simulink model "sampleModel2120_pp"  (R2021a)
settings: Solver=VariableStepAuto  StartTime=0.0  StopTime=10.0  RelTol=1e-3
undefined symbols (not defined in the file or in its folder): DiscIntNeverNeededParam, magnitude, Newton, Raphson
libraries: simulink x67, pid_lib x12
(part 3 of 3)

== system sampleModel2120_pp/cfblk57/cfblk12 ==
  cfblk1 : Inport
  cfblk8 : Inport  Port=2
  cfblk3 : simulink/Discrete/Tapped Delay  vinit=0.0  samptime=-1  NumDelays=1  DelayOrder=Oldest  includeCurrent=off
  cfblk4 : Delay  DelayLengthSource=Input port  SampleTime=1
      settings: InputPortMap=u0,p1
  cfblk5 : Rounding
  cfblk6 : Sin  TimeSource=Use external signal  SampleTime=0
  cfblk7 : Bias  Bias=[-951001195.400587]
  cyemi_{496..501} (6 alike) : DataTypeConversion  OutDataTypeStr=double
  cfblk2 : Outport
  cfblk9 : Outport  Port=2
  wires:
  cfblk7/1 -> cfblk2/1
  cfblk5/1 -> cyemi_496/1, cyemi_498/1
  cfblk4/1 -> cfblk9/1
  cyemi_496/1 -> cfblk3/1
  cyemi_497/1 -> cfblk4/1
  cfblk6/1 -> cyemi_497/1
  cyemi_498/1 -> cfblk4/2
  cyemi_499/1 -> cfblk5/1
  cfblk1/1 -> cyemi_499/1
  cyemi_500/1 -> cfblk6/1
  cfblk3/1 -> cyemi_500/1
  cyemi_501/1 -> cfblk7/1
  cfblk8/1 -> cyemi_501/1

== system sampleModel2120_pp/cfblk57/cfblk13 ==
  cfblk1 : Inport
  cfblk7 : Inport  Port=2
  cfblk3 : simulink/Discrete/Transfer Fcn Real Zero  ZeroZ=0.75  ICPrevInput=0.0  DoSatur=off
      settings: SourceProductBaseCode=SL
  cfblk4 : Sum  Inputs=+-  OutDataTypeStr=double
  cfblk5 : Signum
  cfblk6 : Squeeze
  cyemi_{504..507} (4 alike) : DataTypeConversion  OutDataTypeStr=double
  cfblk2 : Outport
  wires:
  cfblk3/1 -> cfblk6/1
  cfblk6/1 -> cfblk2/1, cyemi_507/1
  cyemi_504/1 -> cfblk3/1
  cfblk4/1 -> cyemi_504/1
  cyemi_505/1 -> cfblk4/1
  cfblk1/1 -> cyemi_505/1
  cyemi_506/1 -> cfblk4/2
  cfblk7/1 -> cyemi_506/1
  cyemi_507/1 -> cfblk5/1

== system sampleModel2120_pp/cfblk57/cfblk14 ==
  cfblk1 : Inport
  cfblk6 : Inport  Port=2
  cfblk3 : Gain  Gain=[374890354.692374]  OutDataTypeStr=double
  cfblk4 : Sqrt  Operator=rSqrt  OutDataTypeStr=double  AlgorithmType=Newton-Raphson  SaturateOnIntegerOverflow=on
  cfblk5 : Product  Inputs=*  OutDataTypeStr=double
  cyemi_510 : DataTypeConversion  OutDataTypeStr=double
  cyemi_511 : DataTypeConversion  OutDataTypeStr=double
  cyemi_512 : DataTypeConversion  OutDataTypeStr=double
  cfblk2 : Outport
  cfblk7 : Outport  Port=2
  cfblk8 : Outport  Port=3
  wires:
  cfblk3/1 -> cfblk7/1
  cfblk1/1 -> cfblk8/1, cyemi_512/1
  cfblk4/1 -> cfblk2/1
  cyemi_510/1 -> cfblk3/1
  cfblk6/1 -> cyemi_510/1
  cyemi_511/1 -> cfblk4/1
  cfblk5/1 -> cyemi_511/1
  cyemi_512/1 -> cfblk5/1

== system sampleModel2120_pp/cfblk57/cfblk15 ==
  cfblk1 : Inport
  cfblk13 : Inport  Port=2
  cfblk14 : Inport  Port=3
  cfblk15 : Inport  Port=4
  cfblk10 : Sin  TimeSource=Use external signal  SampleTime=0
  cfblk11 : UnaryMinus
  cfblk12 : Constant  Value=[495800150.814714]  OutDataTypeStr=double  SampleTime=1
  cfblk3 : simulink/Discrete/Transfer Fcn Real Zero  ZeroZ=0.75  ICPrevInput=0.0  DoSatur=off
      settings: SourceProductBaseCode=SL
  cfblk4 : DiscreteFilter  SampleTime=1
  cfblk5 : simulink/Discrete/Difference  ICPrevInput=0.0  OutMin=[]  OutMax=[]  OutDataTypeStr=double  OutputDataTypeScalingMode=double  OutDataType=fixdt(1, 16)  OutScaling=2^-10  DoSatur=off
  cfblk6 : simulink/Discrete/Transfer Fcn First Order  PoleZ=0.95  ICPrevOutput=0.0  DoSatur=off
  cfblk7 : UnaryMinus
  cfblk8 : MinMax  Inputs=3  OutDataTypeStr=double
  cfblk9 : DotProduct  OutDataTypeStr=double  InputSameDT=on
  cyemi_{517..528} (12 alike) : DataTypeConversion  OutDataTypeStr=double
  cfblk2 : Outport
  cfblk16 : Outport  Port=2
  cfblk17 : Outport  Port=3
  wires:
  cfblk8/1 -> cfblk16/1
  cfblk13/1 -> cfblk2/1
  cfblk10/1 -> cyemi_520/1, cyemi_521/1
  cfblk3/1 -> cfblk17/1
  cyemi_517/1 -> cfblk10/1
  cfblk1/1 -> cyemi_517/1
  cyemi_518/1 -> cfblk11/1
  cfblk15/1 -> cyemi_518/1
  cyemi_519/1 -> cfblk3/1
  cfblk5/1 -> cyemi_519/1
  cyemi_520/1 -> cfblk4/1
  cyemi_521/1 -> cfblk5/1
  cyemi_522/1 -> cfblk6/1
  cfblk9/1 -> cyemi_522/1
  cyemi_523/1 -> cfblk7/1
  cfblk4/1 -> cyemi_523/1
  cyemi_524/1 -> cfblk8/1
  cfblk14/1 -> cyemi_524/1
  cyemi_525/1 -> cfblk8/2
  cfblk6/1 -> cyemi_525/1
  cyemi_526/1 -> cfblk8/3
  cfblk12/1 -> cyemi_526/1
  cyemi_527/1 -> cfblk9/1
  cfblk11/1 -> cyemi_527/1
  cyemi_528/1 -> cfblk9/2
  cfblk7/1 -> cyemi_528/1

== system sampleModel2120_pp/cfblk57/cfblk16 ==
  cfblk1 : Inport
  cfblk13 : Inport  Port=2
  cfblk14 : Inport  Port=3
  cfblk15 : Inport  Port=4
  cfblk16 : Inport  Port=5
  cfblk10 : Abs  OutDataTypeStr=double
  cfblk11 : Sin  TimeSource=Use external signal  SampleTime=0
  cfblk12 : Constant  Value=[868731902.486093]  OutDataTypeStr=double  SampleTime=1
  cfblk3 : simulink/Discrete/Transfer Fcn Real Zero  ZeroZ=0.75  ICPrevInput=0.0  DoSatur=off
      settings: SourceProductBaseCode=SL
  cfblk4 : UnitDelay  HasFrameUpgradeWarning=on
  cfblk5 : Delay  SampleTime=1
  cfblk6 : Trigonometry
  cfblk7 : Sum  Inputs=+-  OutDataTypeStr=double
  cfblk8 : DotProduct  OutDataTypeStr=double  InputSameDT=on
  cfblk9 : Polyval  Coefs=[ +2.081618890e-019, -1.441693666e-014, +4.719686976e-010, -8.536869453e-006, +1.621573104e-001, -8.087801117e+001 ]
  cyemi_{534..544} (11 alike) : DataTypeConversion  OutDataTypeStr=double
  cfblk2 : Outport
  wires:
  cfblk8/1 -> cfblk2/1
  cyemi_534/1 -> cfblk10/1
  cfblk5/1 -> cyemi_534/1
  cyemi_535/1 -> cfblk11/1
  cfblk1/1 -> cyemi_535/1
  cyemi_536/1 -> cfblk3/1
  cfblk4/1 -> cyemi_536/1
  cyemi_537/1 -> cfblk4/1
  cfblk9/1 -> cyemi_537/1
  cyemi_538/1 -> cfblk5/1
  cfblk14/1 -> cyemi_538/1
  cyemi_539/1 -> cfblk6/1
  cfblk11/1 -> cyemi_539/1
  cyemi_540/1 -> cfblk7/1
  cfblk16/1 -> cyemi_540/1
  cyemi_541/1 -> cfblk7/2
  cfblk12/1 -> cyemi_541/1
  cyemi_542/1 -> cfblk8/1
  cfblk7/1 -> cyemi_542/1
  cyemi_543/1 -> cfblk8/2
  cfblk10/1 -> cyemi_543/1
  cyemi_544/1 -> cfblk9/1
  cfblk15/1 -> cyemi_544/1

== system sampleModel2120_pp/cfblk57/cfblk8 ==
  cfblk1 : Inport
  cfblk12 : Inport  Port=2
  cfblk13 : Inport  Port=3
  cfblk10 : Constant  Value=[-135185284.316877]  OutDataTypeStr=double  SampleTime=1
  cfblk11 : Constant  Value=[742840417.275004]  OutDataTypeStr=double  SampleTime=1
  cfblk14 : Delay  SampleTime=1
  cfblk3 : simulink/Discrete/Transfer Fcn Real Zero  ZeroZ=0.75  ICPrevInput=0.0  DoSatur=off
      settings: SourceProductBaseCode=SL
  cfblk4 : simulink/Discrete/Transfer Fcn Real Zero  ZeroZ=0.75  ICPrevInput=0.0  DoSatur=off
      settings: SourceProductBaseCode=SL
  cfblk5 : Delay  ShowEnablePort=on  SampleTime=1
      settings: InputPortMap=u0,e6
  cfblk6 : UnitDelay  HasFrameUpgradeWarning=on
  cfblk7 : Signum
  cfblk8 : DotProduct  OutDataTypeStr=double  InputSameDT=on
  cfblk9 : DotProduct  OutDataTypeStr=double  InputSameDT=on
  cyemi_{558..568} (11 alike) : DataTypeConversion  OutDataTypeStr=double
  cfblk2 : Outport
  wires:
  cfblk12/1 -> cfblk2/1
  cyemi_558/1 -> cfblk14/1
  cfblk8/1 -> cyemi_558/1
  cyemi_559/1 -> cfblk3/1
  cfblk14/1 -> cyemi_559/1
  cyemi_560/1 -> cfblk4/1
  cfblk6/1 -> cyemi_560/1
  cyemi_561/1 -> cfblk5/1
  cfblk1/1 -> cyemi_561/1
  cyemi_562/1 -> cfblk5/2
  cfblk7/1 -> cyemi_562/1
  cyemi_563/1 -> cfblk6/1
  cfblk11/1 -> cyemi_563/1
  cyemi_564/1 -> cfblk7/1
  cfblk13/1 -> cyemi_564/1
  cyemi_565/1 -> cfblk8/1
  cfblk3/1 -> cyemi_565/1
  cyemi_566/1 -> cfblk8/2
  cfblk9/1 -> cyemi_566/1
  cyemi_567/1 -> cfblk9/1
  cfblk4/1 -> cyemi_567/1
  cyemi_568/1 -> cfblk9/2
  cfblk10/1 -> cyemi_568/1

== system sampleModel2120_pp/cfblk57/cfblk9 ==
  cfblk1 : Inport
  cfblk6 : Inport  Port=2
  cfblk3 : DiscreteFilter  SampleTime=1
  cfblk4 : Sqrt  OutDataTypeStr=double  SaturateOnIntegerOverflow=on
  cfblk5 : Constant  Value=[-633278511.677385]  OutDataTypeStr=double  SampleTime=1
  cyemi_571 : DataTypeConversion  OutDataTypeStr=double
  cyemi_572 : DataTypeConversion  OutDataTypeStr=double
  cfblk2 : Outport
  cfblk7 : Outport  Port=2
  wires:
  cfblk4/1 -> cfblk7/1
  cfblk3/1 -> cfblk2/1
  cyemi_571/1 -> cfblk3/1
  cfblk6/1 -> cyemi_571/1
  cyemi_572/1 -> cfblk4/1
  cfblk5/1 -> cyemi_572/1

== system sampleModel2120_pp/cfblk60/cfblk13 ==
  cfblk1 : Inport
  cfblk7 : Inport  Port=2
  cfblk8 : Inport  Port=3
  cfblk9 : Inport  Port=4
  cfblk10 : Delay
  cfblk3 : DotProduct  OutDataTypeStr=double  InputSameDT=on
  cfblk4 : PermuteDimensions
  cfblk5 : DotProduct  OutDataTypeStr=double  InputSameDT=on
  cfblk6 : Signum
  cyemi_{584..590} (7 alike) : DataTypeConversion  OutDataTypeStr=double
  cfblk2 : Outport
  wires:
  cfblk7/1 -> cfblk2/1
  cyemi_584/1 -> cfblk10/1
  cfblk3/1 -> cyemi_584/1
  cyemi_585/1 -> cfblk3/1
  cfblk9/1 -> cyemi_585/1
  cyemi_586/1 -> cfblk3/2
  cfblk4/1 -> cyemi_586/1
  cyemi_587/1 -> cfblk4/1
  cfblk5/1 -> cyemi_587/1
  cyemi_588/1 -> cfblk5/1
  cfblk10/1 -> cyemi_588/1
  cyemi_589/1 -> cfblk5/2
  cfblk1/1 -> cyemi_589/1
  cyemi_590/1 -> cfblk6/1
  cfblk8/1 -> cyemi_590/1

== system sampleModel2120_pp/cfblk61/cfblk10 ==
  cfblk1 : Inport
  cfblk8 : Inport  Port=2
  cfblk9 : Inport  Port=3
  cfblk10 : Inport  Port=4
  cfblk3 : simulink/Discrete/Difference  ICPrevInput=0.0  OutMin=[]  OutMax=[]  OutDataTypeStr=double  OutputDataTypeScalingMode=double  OutDataType=fixdt(1, 16)  OutScaling=2^-10  DoSatur=off
  cfblk4 : pid_lib/PID Controller (2DOF)  Controller=PID  Form=Parallel  TimeDomain=Discrete-time  UseExternalTs=off  SampleTime=-1  IntegratorMethod=Forward Euler  FilterMethod=Forward Euler  ControllerParametersSource=internal  P=1  I=1  D=0  UseFilter=on  N=100  b=1  c=1  TunerSelectOption=Transfer Function Based (PID Tuner App)  InitialConditionSource=internal  InitialConditionForIntegrator=0  InitialConditionForFilter=0  DifferentiatorICPrevScaledInput=0  ExternalReset=none  TrackingMode=off  Kt=1  LimitOutput=off  SatLimitsSource=internal  UpperSaturationLimit=inf  LowerSaturationLimit=-inf  LinearizeAsGain=off  AntiWindupMode=none  Kb=1  POutMin=[]  POutMax=[]  IOutMin=[]  IOutMax=[]  DOutMin=[]  DOutMax=[]  NOutMin=[]  NOutMax=[]  bOutMin=[]  bOutMax=[]  cOutMin=[]  cOutMax=[]  SumOutMin=[]  SumOutMax=[]  SaturationOutMin=[]  SaturationOutMax=[]  PParamMin=[]  PParamMax=[]  IParamMin=[]  IParamMax=[]  DParamMin=[]  DParamMax=[]  NParamMin=[]  NParamMax=[]  bParamMin=[]  bParamMax=[]  cParamMin=[]  cParamMax=[]  KbParamMin=[]  KbParamMax=[]  KtParamMin=[]  KtParamMax=[]  KbOutMin=[]  KbOutMax=[]  KtOutMin=[]  KtOutMax=[]  IntegratorOutMin=[]  IntegratorOutMax=[]  FilterOutMin=[]  FilterOutMax=[]  SumI1OutMin=[]  SumI1OutMax=[]  SumI2OutMin=[]  SumI2OutMax=[]  SumI3OutMin=[]  SumI3OutMax=[]  SumI4OutMin=[]  SumI4OutMax=[]  SumDOutMin=[]  SumDOutMax=[]  Sum1OutMin=[]  Sum1OutMax=[]  Sum2OutMin=[]  Sum2OutMax=[]  Sum3OutMin=[]  Sum3OutMax=[]  DifferentiatorOutMin=[]  DifferentiatorOutMax=[]  FilterDiffOutCoefMin=[]  FilterDiffOutCoefMax=[]  ReciprocalOutMin=[]  ReciprocalOutMax=[]  SumDenOutMin=[]  SumDenOutMax=[]  SumNumOutMin=[]  SumNumOutMax=[]  DivideOutMin=[]  DivideOutMax=[]  UdiffTsProdOutMin=[]  UdiffTsProdOutMax=[]  NTsProdOutMin=[]  NTsProdOutMax=[]  UintegralTsProdOutMin=[]  UintegralTsProdOutMax=[]  UngainTsProdOutMin=[]  UngainTsProdOutMax=[]  IntegratorContinuousStateAttributes=''  IntegratorStateMustResolveToSignalObject=off  IntegratorRTWStateStorageClass=Auto  FilterContinuousStateAttributes=''  FilterStateMustResolveToSignalObject=off  FilterRTWStateStorageClass=Auto  ParallelPVariant=InternalParameters  IdealPVariant=Disabled  IVariant=InternalParameters  DVariant=InternalParameters  bVariant=InternalParameters  cVariant=InternalParameters  IntegratorVariant=Discrete  SatVariant=Disabled  AWVariant=Passthrough  PCopyVariant=Disabled  TRVariant=Disabled  FdbkBlocksVariant=Forward  IdealPFdbkVariant=Disabled  SatFdbkVariant=Disabled  DerivativeFilterVariant=ForwardEulerFilter  NVariant=InternalParameters  NCopyVariant=Disabled  FilterICVariant=InternalICsFilter  IntegratorICVariant=InternalICs  ExternalResetVariant=Disabled  TRSumVariant=Passthrough  SumFdbkVariant=Disabled  SumVariant=Sum_PID  TsampFilterVariant=InternalTs  TsampNgainVariant=Passthrough  TsampIntegralVariant=Passthrough  ExternalSaturationOutDataTypeStr=Inherit: Same as second input
      settings: SourceProductBaseCode=SL
  cfblk5 : Math  Operator=rem  OutDataTypeStr=double  SaturateOnIntegerOverflow=on
  cfblk6 : Constant  Value=[-573577766.807925]  OutDataTypeStr=double  SampleTime=1
  cfblk7 : Constant  Value=[290213308.563316]  OutDataTypeStr=double  SampleTime=1
  cyemi_{612..616} (5 alike) : DataTypeConversion  OutDataTypeStr=double
  cfblk2 : Outport
  wires:
  cfblk3/1 -> cfblk2/1
  cyemi_612/1 -> cfblk3/1
  cfblk8/1 -> cyemi_612/1
  cyemi_613/1 -> cfblk4/1
  cfblk1/1 -> cyemi_613/1
  cyemi_614/1 -> cfblk4/2
  cfblk10/1 -> cyemi_614/1
  cyemi_615/1 -> cfblk5/1
  cfblk9/1 -> cyemi_615/1
  cyemi_616/1 -> cfblk5/2
  cfblk7/1 -> cyemi_616/1

== system sampleModel2120_pp/cfblk61/cfblk11 ==
  cfblk1 : Inport
  cfblk3 : DiscreteTransferFcn
  cfblk4 : DiscreteFir
  cfblk5 : simulink/Discrete/Transfer Fcn Lead or Lag  PoleZ=0.95  ZeroZ=0.75  ICPrevOutput=0.0  ICPrevInput=0.0  DoSatur=off
      settings: SourceProductBaseCode=SL
  cfblk6 : MinMax  Inputs=3  OutDataTypeStr=double
  cfblk8 : Delay
  cyemi_{618..624} (7 alike) : DataTypeConversion  OutDataTypeStr=double
  cfblk2 : Outport
  cfblk7 : Outport  Port=2
  wires:
  cfblk6/1 -> cfblk2/1
  cfblk3/1 -> cfblk7/1, cyemi_622/1
  cfblk4/1 -> cyemi_620/1, cyemi_623/1
  cfblk1/1 -> cyemi_618/1, cyemi_621/1
  cyemi_618/1 -> cfblk3/1
  cyemi_619/1 -> cfblk4/1
  cfblk8/1 -> cyemi_619/1
  cyemi_620/1 -> cfblk5/1
  cyemi_621/1 -> cfblk6/1
  cyemi_622/1 -> cfblk6/2
  cyemi_623/1 -> cfblk6/3
  cyemi_624/1 -> cfblk8/1
  cfblk5/1 -> cyemi_624/1

== system sampleModel2120_pp/cfblk62/cfblk10 ==
  cfblk1 : Inport
  cfblk11 : Inport  Port=2
  cfblk12 : Inport  Port=3
  cfblk13 : Inport  Port=4
  cfblk10 : Constant  Value=[-740955768.227844]  OutDataTypeStr=double  SampleTime=1
  cfblk3 : DiscreteTransferFcn
  cfblk4 : simulink/Discrete/Transfer Fcn Lead or Lag  PoleZ=0.95  ZeroZ=0.75  ICPrevOutput=0.0  ICPrevInput=0.0  DoSatur=off
      settings: SourceProductBaseCode=SL
  cfblk5 : pid_lib/PID Controller (2DOF)  Controller=PID  Form=Parallel  TimeDomain=Discrete-time  UseExternalTs=off  SampleTime=-1  IntegratorMethod=Forward Euler  FilterMethod=Forward Euler  ControllerParametersSource=internal  P=1  I=1  D=0  UseFilter=on  N=100  b=1  c=1  TunerSelectOption=Transfer Function Based (PID Tuner App)  InitialConditionSource=internal  InitialConditionForIntegrator=0  InitialConditionForFilter=0  DifferentiatorICPrevScaledInput=0  ExternalReset=none  TrackingMode=off  Kt=1  LimitOutput=off  SatLimitsSource=internal  UpperSaturationLimit=inf  LowerSaturationLimit=-inf  LinearizeAsGain=off  AntiWindupMode=none  Kb=1  POutMin=[]  POutMax=[]  IOutMin=[]  IOutMax=[]  DOutMin=[]  DOutMax=[]  NOutMin=[]  NOutMax=[]  bOutMin=[]  bOutMax=[]  cOutMin=[]  cOutMax=[]  SumOutMin=[]  SumOutMax=[]  SaturationOutMin=[]  SaturationOutMax=[]  PParamMin=[]  PParamMax=[]  IParamMin=[]  IParamMax=[]  DParamMin=[]  DParamMax=[]  NParamMin=[]  NParamMax=[]  bParamMin=[]  bParamMax=[]  cParamMin=[]  cParamMax=[]  KbParamMin=[]  KbParamMax=[]  KtParamMin=[]  KtParamMax=[]  KbOutMin=[]  KbOutMax=[]  KtOutMin=[]  KtOutMax=[]  IntegratorOutMin=[]  IntegratorOutMax=[]  FilterOutMin=[]  FilterOutMax=[]  SumI1OutMin=[]  SumI1OutMax=[]  SumI2OutMin=[]  SumI2OutMax=[]  SumI3OutMin=[]  SumI3OutMax=[]  SumI4OutMin=[]  SumI4OutMax=[]  SumDOutMin=[]  SumDOutMax=[]  Sum1OutMin=[]  Sum1OutMax=[]  Sum2OutMin=[]  Sum2OutMax=[]  Sum3OutMin=[]  Sum3OutMax=[]  DifferentiatorOutMin=[]  DifferentiatorOutMax=[]  FilterDiffOutCoefMin=[]  FilterDiffOutCoefMax=[]  ReciprocalOutMin=[]  ReciprocalOutMax=[]  SumDenOutMin=[]  SumDenOutMax=[]  SumNumOutMin=[]  SumNumOutMax=[]  DivideOutMin=[]  DivideOutMax=[]  UdiffTsProdOutMin=[]  UdiffTsProdOutMax=[]  NTsProdOutMin=[]  NTsProdOutMax=[]  UintegralTsProdOutMin=[]  UintegralTsProdOutMax=[]  UngainTsProdOutMin=[]  UngainTsProdOutMax=[]  IntegratorContinuousStateAttributes=''  IntegratorStateMustResolveToSignalObject=off  IntegratorRTWStateStorageClass=Auto  FilterContinuousStateAttributes=''  FilterStateMustResolveToSignalObject=off  FilterRTWStateStorageClass=Auto  ParallelPVariant=InternalParameters  IdealPVariant=Disabled  IVariant=InternalParameters  DVariant=InternalParameters  bVariant=InternalParameters  cVariant=InternalParameters  IntegratorVariant=Discrete  SatVariant=Disabled  AWVariant=Passthrough  PCopyVariant=Disabled  TRVariant=Disabled  FdbkBlocksVariant=Forward  IdealPFdbkVariant=Disabled  SatFdbkVariant=Disabled  DerivativeFilterVariant=ForwardEulerFilter  NVariant=InternalParameters  NCopyVariant=Disabled  FilterICVariant=InternalICsFilter  IntegratorICVariant=InternalICs  ExternalResetVariant=Disabled  TRSumVariant=Passthrough  SumFdbkVariant=Disabled  SumVariant=Sum_PID  TsampFilterVariant=InternalTs  TsampNgainVariant=Passthrough  TsampIntegralVariant=Passthrough  ExternalSaturationOutDataTypeStr=Inherit: Same as second input
      settings: SourceProductBaseCode=SL
  cfblk6 : Polyval  Coefs=[ +2.081618890e-019, -1.441693666e-014, +4.719686976e-010, -8.536869453e-006, +1.621573104e-001, -8.087801117e+001 ]
  cfblk7 : Reshape
  cfblk8 : ComplexToRealImag
  cfblk9 : Sum  Inputs=|++  OutDataTypeStr=double
  cyemi_{637..645} (9 alike) : DataTypeConversion  OutDataTypeStr=double
  cfblk2 : Outport
  cfblk14 : Outport  Port=2
  wires:
  cfblk4/1 -> cfblk2/1
  cfblk5/1 -> cfblk14/1
  cyemi_637/1 -> cfblk3/1
  cfblk13/1 -> cyemi_637/1
  cyemi_638/1 -> cfblk4/1
  cfblk7/1 -> cyemi_638/1
  cyemi_639/1 -> cfblk5/1
  cfblk11/1 -> cyemi_639/1
  cyemi_640/1 -> cfblk5/2
  cfblk1/1 -> cyemi_640/1
  cyemi_641/1 -> cfblk6/1
  cfblk3/1 -> cyemi_641/1
  cyemi_642/1 -> cfblk7/1
  cfblk8/1 -> cyemi_642/1
  cyemi_643/1 -> cfblk8/1
  cfblk9/1 -> cyemi_643/1
  cyemi_644/1 -> cfblk9/1
  cfblk6/1 -> cyemi_644/1
  cyemi_645/1 -> cfblk9/2
  cfblk10/1 -> cyemi_645/1

== system sampleModel2120_pp/cfblk62/cfblk11 ==
  cfblk1 : Inport
  cfblk7 : Inport  Port=2
  cfblk8 : Inport  Port=3
  cfblk3 : Sum  Inputs=+-  OutDataTypeStr=double
  cfblk4 : Bias  Bias=[-682721005.322066]
  cfblk5 : Product  OutDataTypeStr=double
  cfblk6 : PermuteDimensions
  cfblk9 : Delay
  cyemi_{649..655} (7 alike) : DataTypeConversion  OutDataTypeStr=double
  cfblk2 : Outport
  wires:
  cfblk5/1 -> cfblk2/1
  cyemi_649/1 -> cfblk3/1
  cfblk4/1 -> cyemi_649/1
  cyemi_650/1 -> cfblk3/2
  cfblk9/1 -> cyemi_650/1
  cyemi_651/1 -> cfblk4/1
  cfblk7/1 -> cyemi_651/1
  cyemi_652/1 -> cfblk5/1
  cfblk1/1 -> cyemi_652/1
  cyemi_653/1 -> cfblk5/2
  cfblk8/1 -> cyemi_653/1
  cyemi_654/1 -> cfblk6/1
  cfblk3/1 -> cyemi_654/1
  cyemi_655/1 -> cfblk9/1
  cfblk6/1 -> cyemi_655/1

== system sampleModel2120_pp/cfblk62/cfblk14 ==
  cfblk1 : Inport
  cfblk7 : Inport  Port=2
  Action Port : ActionPort  ActionPortLabel=if(u1 >= 0)
  cfblk3 : Squeeze
  cfblk4 : Product  Inputs=*  OutDataTypeStr=double
  cfblk5 : Sqrt  OutDataTypeStr=double  SaturateOnIntegerOverflow=on
  cfblk6 : Math  Operator=square  OutDataTypeStr=double  SaturateOnIntegerOverflow=on
  cyemi_659 : DataTypeConversion  OutDataTypeStr=double
  cyemi_660 : DataTypeConversion  OutDataTypeStr=double
  cyemi_661 : DataTypeConversion  OutDataTypeStr=double
  cfblk2 : Outport
  cfblk8 : Outport  Port=2
  wires:
  cfblk7/1 -> cfblk3/1
  cfblk6/1 -> cfblk8/1
  cfblk1/1 -> cfblk2/1
  cyemi_659/1 -> cfblk4/1
  cfblk5/1 -> cyemi_659/1
  cyemi_660/1 -> cfblk5/1
  cfblk3/1 -> cyemi_660/1
  cyemi_661/1 -> cfblk6/1
  cfblk4/1 -> cyemi_661/1

== system sampleModel2120_pp/cfblk62/cfblk15 ==
  cfblk1 : Inport
  Action Port : ActionPort  ActionPortLabel=else
  cfblk3 : pid_lib/PID Controller  Controller=PID  Form=Parallel  TimeDomain=Discrete-time  UseExternalTs=off  SampleTime=-1  IntegratorMethod=Forward Euler  FilterMethod=Forward Euler  ControllerParametersSource=internal  P=1  I=1  D=0  UseFilter=on  N=100  TunerSelectOption=Transfer Function Based (PID Tuner App)  InitialConditionSource=internal  InitialConditionForIntegrator=0  InitialConditionForFilter=0  DifferentiatorICPrevScaledInput=0  ExternalReset=none  TrackingMode=off  Kt=1  LimitOutput=off  SatLimitsSource=internal  UpperSaturationLimit=inf  LowerSaturationLimit=-inf  LinearizeAsGain=off  AntiWindupMode=none  Kb=1  POutMin=[]  POutMax=[]  IOutMin=[]  IOutMax=[]  DOutMin=[]  DOutMax=[]  NOutMin=[]  NOutMax=[]  SumOutMin=[]  SumOutMax=[]  SaturationOutMin=[]  SaturationOutMax=[]  PParamMin=[]  PParamMax=[]  IParamMin=[]  IParamMax=[]  DParamMin=[]  DParamMax=[]  NParamMin=[]  NParamMax=[]  KbParamMin=[]  KbParamMax=[]  KtParamMin=[]  KtParamMax=[]  KbOutMin=[]  KbOutMax=[]  KtOutMin=[]  KtOutMax=[]  IntegratorOutMin=[]  IntegratorOutMax=[]  FilterOutMin=[]  FilterOutMax=[]  SumI1OutMin=[]  SumI1OutMax=[]  SumI2OutMin=[]  SumI2OutMax=[]  SumI3OutMin=[]  SumI3OutMax=[]  SumI4OutMin=[]  SumI4OutMax=[]  SumDOutMin=[]  SumDOutMax=[]  DifferentiatorOutMin=[]  DifferentiatorOutMax=[]  FilterDiffOutCoefMin=[]  FilterDiffOutCoefMax=[]  ReciprocalOutMin=[]  ReciprocalOutMax=[]  SumDenOutMin=[]  SumDenOutMax=[]  SumNumOutMin=[]  SumNumOutMax=[]  DivideOutMin=[]  DivideOutMax=[]  UdiffTsProdOutMin=[]  UdiffTsProdOutMax=[]  NTsProdOutMin=[]  NTsProdOutMax=[]  UintegralTsProdOutMin=[]  UintegralTsProdOutMax=[]  UngainTsProdOutMin=[]  UngainTsProdOutMax=[]  IntegratorContinuousStateAttributes=''  IntegratorStateMustResolveToSignalObject=off  IntegratorRTWStateStorageClass=Auto  FilterContinuousStateAttributes=''  FilterStateMustResolveToSignalObject=off  FilterRTWStateStorageClass=Auto  ParallelPVariant=InternalParameters  IdealPVariant=Disabled  IVariant=InternalParameters  DVariant=InternalParameters  IntegratorVariant=Discrete  SatVariant=Disabled  AWVariant=Passthrough  PCopyVariant=Disabled  TRVariant=Disabled  FdbkBlocksVariant=Forward  IdealPFdbkVariant=Disabled  SatFdbkVariant=Disabled  DerivativeFilterVariant=ForwardEulerFilter  NVariant=InternalParameters  NCopyVariant=Disabled  FilterICVariant=InternalICsFilter  IntegratorICVariant=InternalICs  ExternalResetVariant=Disabled  TRSumVariant=Passthrough  SumFdbkVariant=Disabled  SumVariant=Sum_PID  TsampFilterVariant=InternalTs  TsampNgainVariant=Passthrough  TsampIntegralVariant=Passthrough  ExternalSaturationOutDataTypeStr=Inherit: Same as second input
  cfblk4 : ComplexToMagnitudeAngle
  cfblk5 : ComplexToMagnitudeAngle
  cfblk6 : simulink/Math Operations/Slider Gain  gain=1  low=0  high=2
  cfblk7 : Abs  OutDataTypeStr=double
  cyemi_{663..667} (5 alike) : DataTypeConversion  OutDataTypeStr=double
  cfblk2 : Outport
  wires:
  cfblk7/1 -> cfblk2/1
  cyemi_663/1 -> cfblk3/1
  cfblk4/1 -> cyemi_663/1
  cyemi_664/1 -> cfblk4/1
  cfblk6/1 -> cyemi_664/1
  cyemi_665/1 -> cfblk5/1
  cfblk3/1 -> cyemi_665/1
  cyemi_666/1 -> cfblk6/1
  cfblk1/1 -> cyemi_666/1
  cyemi_667/1 -> cfblk7/1
  cfblk5/1 -> cyemi_667/1

== system sampleModel2120_pp/cfblk62/cfblk9 ==
  cfblk1 : Inport
  cfblk10 : Inport  Port=2
  cfblk11 : Inport  Port=3
  cfblk13 : Delay
  cfblk14 : Delay
  cfblk3 : Delay  DelayLengthSource=Input port
      settings: InputPortMap=u0,p1
  cfblk4 : simulink/Discrete/Transfer Fcn Lead or Lag  PoleZ=0.95  ZeroZ=0.75  ICPrevOutput=0.0  ICPrevInput=0.0  DoSatur=off
      settings: SourceProductBaseCode=SL
  cfblk5 : simulink/Discrete/Transfer Fcn Real Zero  ZeroZ=0.75  ICPrevInput=0.0  DoSatur=off
      settings: SourceProductBaseCode=SL
  cfblk6 : Polyval  Coefs=[ +2.081618890e-019, -1.441693666e-014, +4.719686976e-010, -8.536869453e-006, +1.621573104e-001, -8.087801117e+001 ]
  cfblk7 : MinMax  Function=max  OutDataTypeStr=double
  cfblk8 : simulink/Math Operations/MinMax Running Resettable  Function=min  vinit=0.0
  cfblk9 : Sum  Inputs=|++  OutDataTypeStr=double
  cyemi_{683..694} (12 alike) : DataTypeConversion  OutDataTypeStr=double
  cfblk2 : Outport
  cfblk12 : Outport  Port=2
  wires:
  cfblk8/1 -> cfblk2/1, cyemi_684/1
  cfblk6/1 -> cfblk12/1
  cfblk3/1 -> cyemi_690/1, cyemi_692/1
  cyemi_683/1 -> cfblk13/1
  cfblk7/1 -> cyemi_683/1
  cyemi_684/1 -> cfblk14/1
  cyemi_685/1 -> cfblk3/1
  cfblk14/1 -> cyemi_685/1
  cyemi_686/1 -> cfblk3/2
  cfblk9/1 -> cyemi_686/1
  cyemi_687/1 -> cfblk4/1
  cfblk11/1 -> cyemi_687/1
  cyemi_688/1 -> cfblk5/1
  cfblk1/1 -> cyemi_688/1
  cyemi_689/1 -> cfblk6/1
  cfblk4/1 -> cyemi_689/1
  cyemi_690/1 -> cfblk7/1
  cyemi_691/1 -> cfblk8/1
  cfblk10/1 -> cyemi_691/1
  cyemi_692/1 -> cfblk8/2
  cyemi_693/1 -> cfblk9/1
  cfblk5/1 -> cyemi_693/1
  cyemi_694/1 -> cfblk9/2
  cfblk13/1 -> cyemi_694/1

== system sampleModel2120_pp/cfblk63/cfblk7 ==
  cfblk1 : Inport
  cfblk9 : Inport  Port=2
  cfblk10 : Inport  Port=3
  cfblk3 : simulink/Discrete/Transfer Fcn Lead or Lag  PoleZ=0.95  ZeroZ=0.75  ICPrevOutput=0.0  ICPrevInput=0.0  DoSatur=off
      settings: SourceProductBaseCode=SL
  cfblk4 : Bias  Bias=[735508419.824777]
  cfblk5 : Sum  Inputs=+-  OutDataTypeStr=double
  cfblk6 : Signum
  cfblk7 : Product  OutDataTypeStr=double
  cfblk8 : Constant  Value=[-371589237.003907]  OutDataTypeStr=double  SampleTime=1
  cyemi_{707..713} (7 alike) : DataTypeConversion  OutDataTypeStr=double
  cfblk2 : Outport
  cfblk11 : Outport  Port=2
  cfblk12 : Outport  Port=3
  wires:
  cfblk4/1 -> cfblk12/1
  cfblk5/1 -> cyemi_707/1, cyemi_712/1
  cfblk9/1 -> cfblk2/1
  cfblk10/1 -> cfblk11/1
  cyemi_707/1 -> cfblk3/1
  cyemi_708/1 -> cfblk4/1
  cfblk7/1 -> cyemi_708/1
  cyemi_709/1 -> cfblk5/1
  cfblk6/1 -> cyemi_709/1
  cyemi_710/1 -> cfblk5/2
  cfblk1/1 -> cyemi_710/1
  cyemi_711/1 -> cfblk6/1
  cfblk8/1 -> cyemi_711/1
  cyemi_712/1 -> cfblk7/1
  cyemi_713/1 -> cfblk7/2
  cfblk3/1 -> cyemi_713/1
